simulink model "model2"  (R2022a)
settings: Solver=VariableStepAuto  StartTime=0.0  StopTime=0.4  RelTol=1e-3
values from neighbouring files (symbols this model uses):
  K = H/M    [tasks.m]
  T = 0.005    [config.m]
  W_1 = K_1/(Tau_1*s + 1)    [config.m]
  W_2 = K_2/(Tau_2*s + 1)    [config.m]
  W_3 = K_3/s    [config.m]
settings Model: Creator=Vvlad  LastModifiedBy=Vvlad

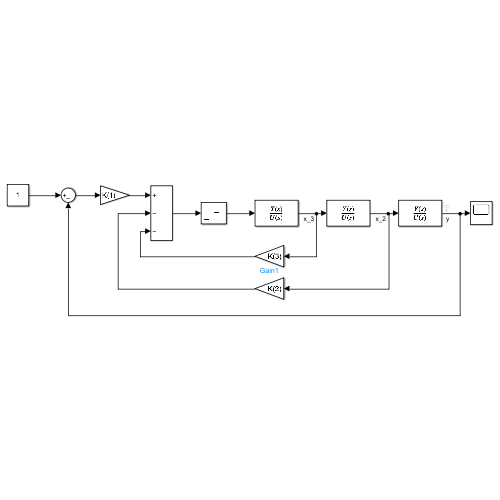
[thumbnail: Simulink's stored preview of the top-level diagram]
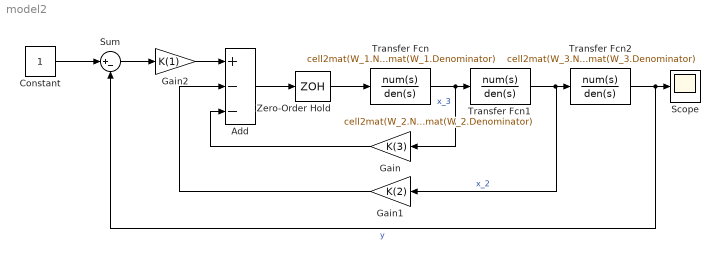
== system model2 ==
  Add : Sum  Inputs=+--
  Constant : Constant
  Gain : Gain  Gain=K(3)
  Gain1 : Gain  Gain=K(2)
  Gain2 : Gain  Gain=K(1)
  Scope : Scope
  Sum : Sum  Inputs=|+-
  Transfer Fcn : TransferFcn  Numerator=cell2mat(W_1.Numerator)  Denominator=cell2mat(W_1.Denominator)
  Transfer Fcn1 : TransferFcn  Numerator=cell2mat(W_2.Numerator)  Denominator=cell2mat(W_2.Denominator)
  Transfer Fcn2 : TransferFcn  Numerator=cell2mat(W_3.Numerator)  Denominator=cell2mat(W_3.Denominator)
  Zero-Order Hold : ZeroOrderHold  SampleTime=T
  wires:
  Transfer Fcn1/1 -> Gain1/1, Transfer Fcn2/1  "x_2"
  Transfer Fcn/1 -> Gain/1, Transfer Fcn1/1  "x_3"
  Zero-Order Hold/1 -> Transfer Fcn/1
  Transfer Fcn2/1 -> Sum/2, Scope/1  "y"
  Sum/1 -> Gain2/1
  Add/1 -> Zero-Order Hold/1
  Gain/1 -> Add/3
  Gain1/1 -> Add/2
  Constant/1 -> Sum/1
  Gain2/1 -> Add/1
